simulink subsystem "mashine"  (R2023a)
settings: Solver=VariableStepAuto  StartTime=0.0  StopTime=10.0  RelTol=1e-3
model mask{k=7, T1=0.1, T2=0.05}
  mask prompts: k "Коэффициент усиления"; T1 "(Частота переключения 1)^-1"; T2 "(Частота переключения 2)^-1"
settings Model: Creator=diontep  LastModifiedBy=diontep

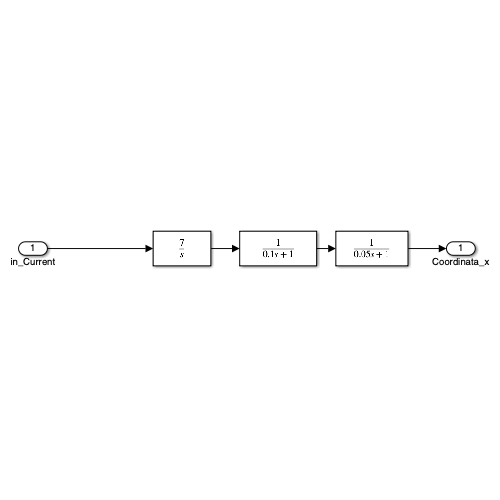
[thumbnail: Simulink's stored preview of the top-level diagram]
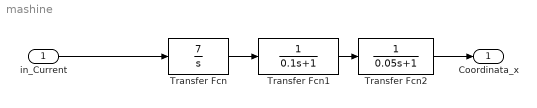
== system mashine ==
  in_Current : Inport
  Transfer Fcn : TransferFcn  Numerator=[7]  Denominator=[1 0]
  Transfer Fcn1 : TransferFcn  Denominator=[0.1 1]
  Transfer Fcn2 : TransferFcn  Denominator=[0.05 1]
  Coordinata_x : Outport
  wires:
  Transfer Fcn1/1 -> Transfer Fcn2/1
  Transfer Fcn/1 -> Transfer Fcn1/1
  in_Current/1 -> Transfer Fcn/1
  Transfer Fcn2/1 -> Coordinata_x/1
